simulink model "Signal_modulant"  (R2021a)
settings: Solver=FixedStepDiscrete  StartTime=0.0  StopTime=10e-3  FixedStep=1e-6  RelTol=1e-3
libraries: dspsrcs4 x3
settings Model: Creator=jimmypan  LastModifiedBy=jimmypan

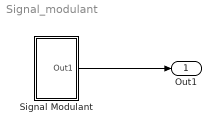
== system Signal_modulant ==
  Signal Modulant : Subsystem
  Out1 : Outport
  wires:
  Signal Modulant/1(Out1) -> Out1/1

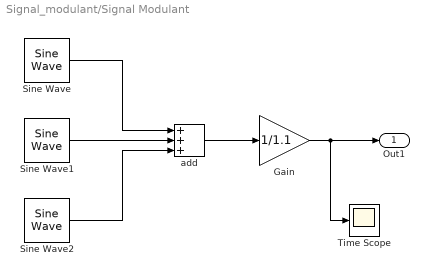
== system Signal_modulant/Signal Modulant ==
  Gain : Gain  Gain=1/1.1
  Sine Wave : dspsrcs4/Sine Wave  Amplitude=1  Frequency=500  Phase=0  SampleMode=Discrete  OutComplex=Real  CompMethod=Trigonometric fcn  TableSize=Speed  SampleTime=1/1000000  SamplesPerFrame=1  ResetState=Restart at time zero  OutputFrames=off  dataType=double  wordLen=16  udDataType=sfix(16)  fracBitsMode=Best precision  numFracBits=15  OutDataTypeStr=double  LastOutDataTypeStr=double
  Sine Wave1 : dspsrcs4/Sine Wave  Amplitude=0.5  Frequency=1500  Phase=0  SampleMode=Discrete  OutComplex=Real  CompMethod=Trigonometric fcn  TableSize=Speed  SampleTime=1/1000000  SamplesPerFrame=1  ResetState=Restart at time zero  OutputFrames=off  dataType=double  wordLen=16  udDataType=sfix(16)  fracBitsMode=Best precision  numFracBits=15  OutDataTypeStr=double  LastOutDataTypeStr=double
  Sine Wave2 : dspsrcs4/Sine Wave  Amplitude=0.2  Frequency=2500  Phase=0  SampleMode=Discrete  OutComplex=Real  CompMethod=Trigonometric fcn  TableSize=Speed  SampleTime=1/1000000  SamplesPerFrame=1  ResetState=Restart at time zero  OutputFrames=off  dataType=double  wordLen=16  udDataType=sfix(16)  fracBitsMode=Best precision  numFracBits=15  OutDataTypeStr=double  LastOutDataTypeStr=double
  Time Scope : Scope
  add : Sum  Inputs=+++
  Out1 : Outport
  wires:
  add/1 -> Gain/1
  Sine Wave2/1 -> add/3
  Sine Wave/1 -> add/1
  Sine Wave1/1 -> add/2
  Gain/1 -> Out1/1, Time Scope/1
